simulink subsystem "ILYA_Subsystem"  (R2023b)
settings: Solver=VariableStepAuto  StartTime=0.0  StopTime=10.0  RelTol=1e-3
settings Model: Creator=diontep  LastModifiedBy=a2

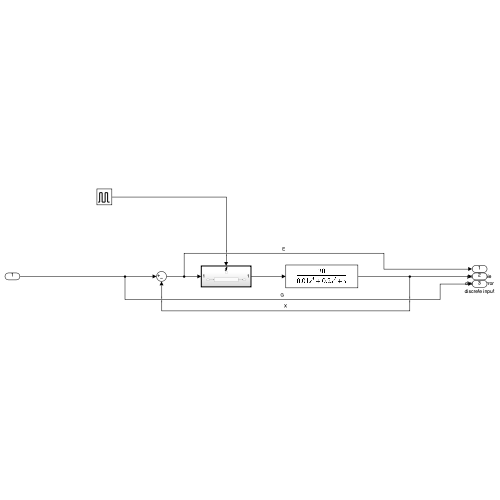
[thumbnail: Simulink's stored preview of the top-level diagram]
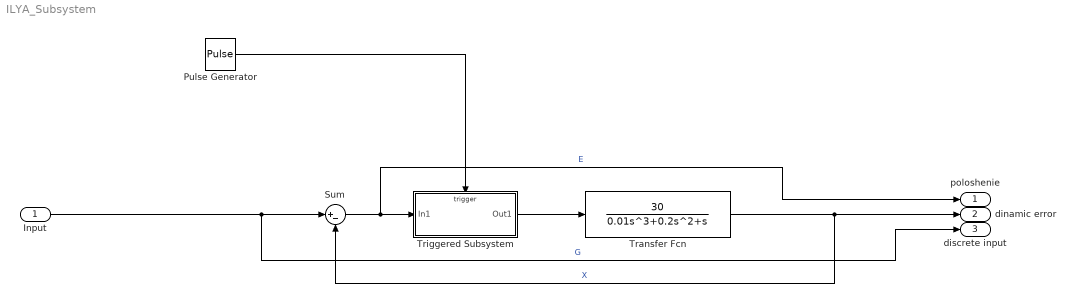
== system ILYA_Subsystem ==
  Input : Inport
  Pulse Generator : DiscretePulseGenerator  PulseType=Time based  Period=0.005  PulseWidth=5
  Sum : Sum  Inputs=|+-
  Transfer Fcn : TransferFcn  Numerator=[30]  Denominator=[0.01 0.2 1 0]
  Triggered Subsystem : Subsystem  TreatAsAtomicUnit=on
  poloshenie : Outport
  dinamic error : Outport  Port=2
  discrete input : Outport  Port=3
  wires:
  Sum/1 -> poloshenie/1, Triggered Subsystem/1(In1)  "E"
  Input/1 -> discrete input/1, Sum/1  "G"
  Transfer Fcn/1 -> dinamic error/1, Sum/2  "X"
  Triggered Subsystem/1(Out1) -> Transfer Fcn/1
  Pulse Generator/1 -> Triggered Subsystem/Trigger

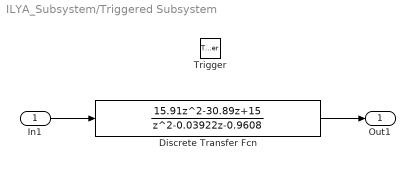
== system ILYA_Subsystem/Triggered Subsystem ==
  In1 : Inport
  Trigger : TriggerPort  VariantControl=(inherit)
  Discrete Transfer Fcn : DiscreteTransferFcn  Numerator=[15.91 -30.89 15]  Denominator=[1 -0.03922 -0.9608]
  Out1 : Outport
  wires:
  Discrete Transfer Fcn/1 -> Out1/1
  In1/1 -> Discrete Transfer Fcn/1
